simulink model "sim_model"  (R2019b)
settings: Solver=VariableStepAuto  StartTime=0.0  StopTime=10.0  MaxStep=0.0001  RelTol=1e-3
values from neighbouring files (symbols this model uses):
  A_et = conv([16*Tu 1], [4*Tu 1])    [astatism.m]    (also in binomial.m = [1]; linear_opt.m = [1]; symmetrical.m = [4*Tu 1]; technical.m = [1])
  A_ou = [Kob]    [astatism.m]    (also in binomial.m; linear_opt.m = [1]; symmetrical.m; technical.m = [1])
  A_r = conv(conv([T1 1], [16*Tu 1]), [4*Tu 1])    [astatism.m]    (also in binomial.m = [T1 1]; linear_opt.m = [T1 1]; symmetrical.m = conv([4*Tu 1], [T1 1]); technical.m = [T1 1])
  B_et = [128*Tu^4 128*Tu^3 64*Tu^2 20*Tu 1]    [astatism.m]    (also in binomial.m = [3*Tu^2 3*Tu 1]; linear_opt.m = [T2 1]; symmetrical.m = [8*Tu^3 8*Tu^2 4*Tu 1]; technical.m = [2*Tu^2 2*Tu 1])
  B_ou = conv([T1 1], [T2 1 0])    [astatism.m]    (also in binomial.m = conv([T1 1], [T2 1]); linear_opt.m = [T1 1]; symmetrical.m = conv(conv([T1 1], [T2 1]), [1 0]); technical.m = conv([T1 1], [T2 1]))
  B_r = conv(B_r, [0.00001 1])    [astatism.m]    (also in binomial.m = [3*Tu*Kob 0]; linear_opt.m = [T2 0]; symmetrical.m; technical.m = [2*Tu 0])
settings Model: Creator=yktma  LastModifiedBy=yktma
settings DataIOCC: ExternalInput=signal  LoadExternalInput=on

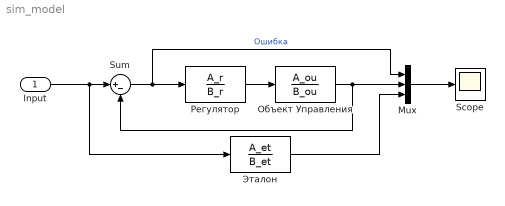
== system sim_model ==
  Input : Inport
  Mux : Mux  Inputs=3
  Scope : Scope
  Sum : Sum  Inputs=|+-
  Объект Управления : TransferFcn  Numerator=A_ou  Denominator=B_ou
  Регулятор : TransferFcn  Numerator=A_r  Denominator=B_r
  Эталон : TransferFcn  Numerator=A_et  Denominator=B_et
  wires:
  Input/1 -> Эталон/1, Sum/1
  Sum/1 -> Mux/1, Регулятор/1  "Ошибка"
  Регулятор/1 -> Объект Управления/1
  Эталон/1 -> Mux/3
  Объект Управления/1 -> Sum/2, Mux/2
  Mux/1 -> Scope/1
